simulink model "Star"  (R2022a)
settings: Solver=VariableStepAuto  StartTime=0.0  StopTime=10.0  RelTol=1e-3
undefined symbols (not defined in the file or in its folder): magnitude
libraries: commchan3 x1
settings Model: Creator=emmamarsden  LastModifiedBy=emmamarsden

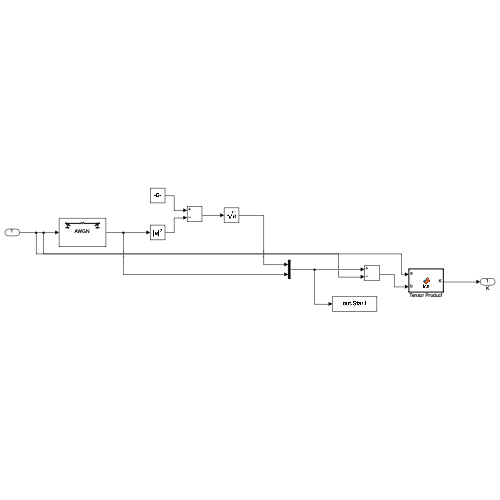
[thumbnail: Simulink's stored preview of the top-level diagram]
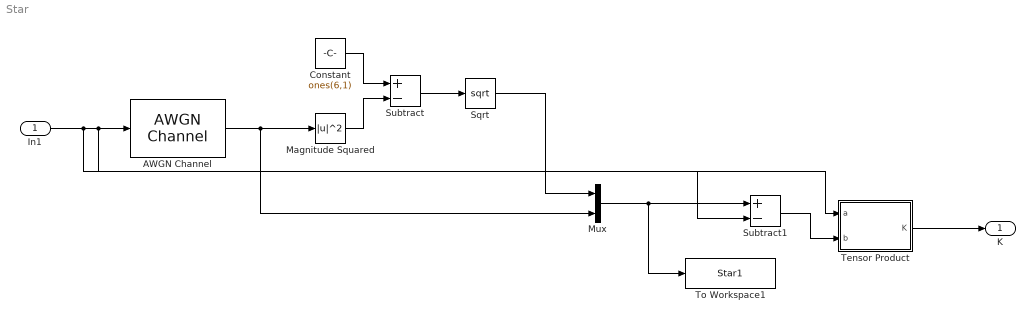
== system Star ==
  In1 : Inport
  AWGN Channel : commchan3/AWGN Channel  InputProcessing=Columns as channels (frame based)  seed=67  noiseMode="Signal to noise ratio  (Eb/No)"  EbNodB=10  EsNodB=10  SNRdB=10  bitsPerSym=1  Ps=1  Tsym=1  variance=1
  Constant : Constant  Value=ones(6,1)
  Magnitude Squared : Math  Operator=magnitude^2
  Mux : Mux  Inputs=2
  Sqrt : Sqrt
  Subtract : Sum  Inputs=+-
  Subtract1 : Sum  Inputs=+-
  Tensor Product : MATLAB Function  TreatAsAtomicUnit=on
  To Workspace1 : ToWorkspace  VariableName=Star1  SaveFormat=Timeseries  SampleTime=-1
  K : Outport
  wires:
  Tensor Product/1(K) -> K/1
  Subtract1/1 -> Tensor Product/2(b)
  Mux/1 -> To Workspace1/1, Subtract1/1
  Sqrt/1 -> Mux/1
  Magnitude Squared/1 -> Subtract/2
  Subtract/1 -> Sqrt/1
  AWGN Channel/1 -> Magnitude Squared/1, Mux/2
  Constant/1 -> Subtract/1
  In1/1 -> Subtract1/2, Tensor Product/1(a), AWGN Channel/1

== matlab function Star/Tensor Product ==
  data: a input; K output; b input
function K = fcn(a,b)

K = kron(a,b);
